simulink model "Vehicle10DOF"  (R2026b)
settings: Solver=ode45  StopTime=1
undefined symbols (not defined in the file): Tire, Vehicle, Vehicle7DOFInitialState
settings Model: DataDictionary=VehicleData.sldd  Creator=Xu Dingyi  LastModifiedBy=29358
settings ModelReferenceCC: ModelReferenceMinAlgLoopOccurrences=on

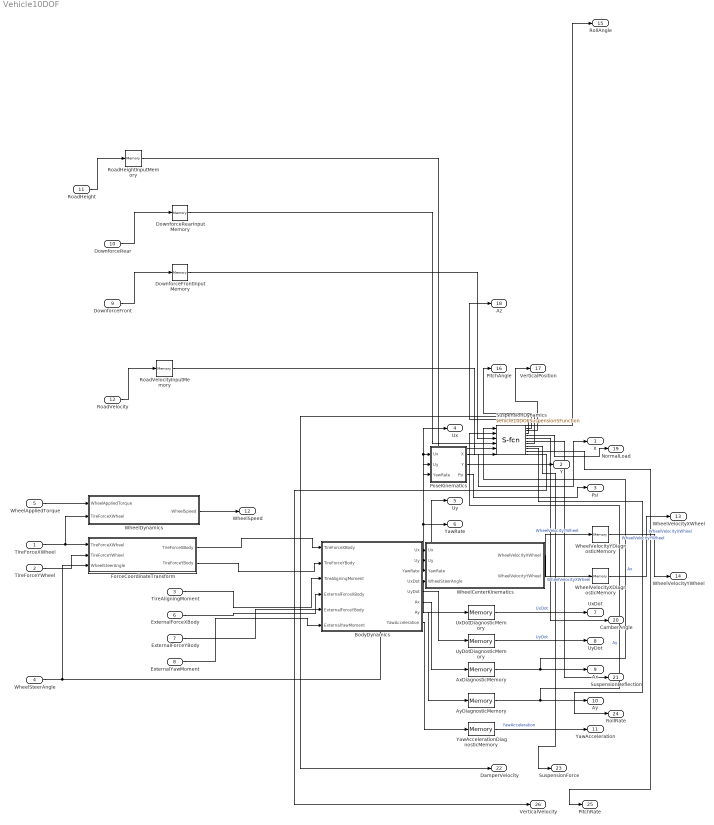
== system Vehicle10DOF ==
  TireForceXWheel : Inport  OutDataTypeStr=double  PortDimensions=[4 1]
  TireForceYWheel : Inport  Port=2  OutDataTypeStr=double  PortDimensions=[4 1]
  TireAligningMoment : Inport  Port=3  OutDataTypeStr=double  PortDimensions=[4 1]
  WheelSteerAngle : Inport  Port=4  OutDataTypeStr=double  PortDimensions=[4 1]
  WheelAppliedTorque : Inport  Port=5  OutDataTypeStr=double  PortDimensions=[4 1]
  ExternalForceXBody : Inport  Port=6  OutDataTypeStr=double  PortDimensions=1
  ExternalForceYBody : Inport  Port=7  OutDataTypeStr=double  PortDimensions=1
  ExternalYawMoment : Inport  Port=8  OutDataTypeStr=double  PortDimensions=1
  DownforceFront : Inport  Port=9
  DownforceRear : Inport  Port=10
  RoadHeight : Inport  Port=11  PortDimensions=4
  RoadVelocity : Inport  Port=12  PortDimensions=4
  AxDiagnosticMemory : Memory
  AyDiagnosticMemory : Memory
  BodyDynamics : Subsystem
  DownforceFrontInputMemory : Memory
  DownforceRearInputMemory : Memory
  ForceCoordinateTransform : Subsystem
  PoseKinematics : Subsystem
  RoadHeightInputMemory : Memory
  RoadVelocityInputMemory : Memory
  SuspensionDynamics : M-S-Function  FunctionName=vehicle10DOFSuspensionSFunction  Parameters=Vehicle10DOFSuspension
  UxDotDiagnosticMemory : Memory
  UyDotDiagnosticMemory : Memory
  WheelCenterKinematics : Subsystem
  WheelDynamics : Subsystem
  WheelVelocityXDiagnosticMemory : Memory
  WheelVelocityYDiagnosticMemory : Memory
  YawAccelerationDiagnosticMemory : Memory
  X : Outport
  Y : Outport  Port=2
  Psi : Outport  Port=3
  Ux : Outport  Port=4
  Uy : Outport  Port=5
  YawRate : Outport  Port=6
  UxDot : Outport  Port=7
  UyDot : Outport  Port=8
  Ax : Outport  Port=9
  Ay : Outport  Port=10
  YawAcceleration : Outport  Port=11
  WheelSpeed : Outport  Port=12
  WheelVelocityXWheel : Outport  Port=13
  WheelVelocityYWheel : Outport  Port=14
  RollAngle : Outport  Port=15
  PitchAngle : Outport  Port=16
  VerticalPosition : Outport  Port=17
  Az : Outport  Port=18
  NormalLoad : Outport  Port=19
  CamberAngle : Outport  Port=20
  SuspensionDeflection : Outport  Port=21
  DamperVelocity : Outport  Port=22
  SuspensionForce : Outport  Port=23
  RollRate : Outport  Port=24
  PitchRate : Outport  Port=25
  VerticalVelocity : Outport  Port=26
  wires:
  WheelSteerAngle/1 -> WheelCenterKinematics/4(WheelSteerAngle), ForceCoordinateTransform/3(WheelSteerAngle)
  TireForceYWheel/1 -> ForceCoordinateTransform/2(TireForceYWheel)
  TireForceXWheel/1 -> ForceCoordinateTransform/1(TireForceXWheel), WheelDynamics/2(TireForceXWheel)
  WheelAppliedTorque/1 -> WheelDynamics/1(WheelAppliedTorque)
  YawAccelerationDiagnosticMemory/1 -> YawAcceleration/1  "YawAcceleration"
  WheelDynamics/1(WheelSpeed) -> WheelSpeed/1
  UxDotDiagnosticMemory/1 -> UxDot/1  "UxDot"
  UyDotDiagnosticMemory/1 -> UyDot/1  "UyDot"
  AyDiagnosticMemory/1 -> SuspensionDynamics/2, Ay/1  "Ay"
  ForceCoordinateTransform/1(TireForceXBody) -> BodyDynamics/1(TireForceXBody)
  ForceCoordinateTransform/2(TireForceYBody) -> BodyDynamics/2(TireForceYBody)
  TireAligningMoment/1 -> BodyDynamics/3(TireAligningMoment)
  ExternalForceXBody/1 -> BodyDynamics/4(ExternalForceXBody)
  ExternalForceYBody/1 -> BodyDynamics/5(ExternalForceYBody)
  ExternalYawMoment/1 -> BodyDynamics/6(ExternalYawMoment)
  BodyDynamics/4(UxDot) -> UxDotDiagnosticMemory/1
  BodyDynamics/5(UyDot) -> UyDotDiagnosticMemory/1
  BodyDynamics/6(Ax) -> AxDiagnosticMemory/1
  BodyDynamics/7(Ay) -> AyDiagnosticMemory/1
  BodyDynamics/8(YawAcceleration) -> YawAccelerationDiagnosticMemory/1
  AxDiagnosticMemory/1 -> SuspensionDynamics/1, Ax/1  "Ax"
  BodyDynamics/1(Ux) -> Ux/1, PoseKinematics/1(Ux), WheelCenterKinematics/1(Ux)
  BodyDynamics/2(Uy) -> PoseKinematics/2(Uy), Uy/1, WheelCenterKinematics/2(Uy)
  BodyDynamics/3(YawRate) -> PoseKinematics/3(YawRate), YawRate/1, WheelCenterKinematics/3(YawRate)
  PoseKinematics/1(X) -> X/1
  PoseKinematics/2(Y) -> Y/1
  PoseKinematics/3(Psi) -> Psi/1
  WheelCenterKinematics/1(WheelVelocityXWheel) -> WheelVelocityXDiagnosticMemory/1  "WheelVelocityXWheel"
  WheelVelocityXDiagnosticMemory/1 -> WheelVelocityXWheel/1  "WheelVelocityXWheel"
  WheelCenterKinematics/2(WheelVelocityYWheel) -> WheelVelocityYDiagnosticMemory/1  "WheelVelocityYWheel"
  WheelVelocityYDiagnosticMemory/1 -> WheelVelocityYWheel/1  "WheelVelocityYWheel"
  DownforceFront/1 -> DownforceFrontInputMemory/1
  DownforceRear/1 -> DownforceRearInputMemory/1
  RoadHeight/1 -> RoadHeightInputMemory/1
  RoadVelocity/1 -> RoadVelocityInputMemory/1
  SuspensionDynamics/1 -> RollAngle/1
  SuspensionDynamics/2 -> PitchAngle/1
  SuspensionDynamics/3 -> VerticalPosition/1
  SuspensionDynamics/4 -> Az/1
  SuspensionDynamics/5 -> NormalLoad/1
  SuspensionDynamics/6 -> CamberAngle/1
  SuspensionDynamics/7 -> SuspensionDeflection/1
  SuspensionDynamics/8 -> DamperVelocity/1
  SuspensionDynamics/9 -> SuspensionForce/1
  SuspensionDynamics/10 -> RollRate/1
  SuspensionDynamics/11 -> PitchRate/1
  SuspensionDynamics/12 -> VerticalVelocity/1
  DownforceFrontInputMemory/1 -> SuspensionDynamics/3
  DownforceRearInputMemory/1 -> SuspensionDynamics/4
  RoadHeightInputMemory/1 -> SuspensionDynamics/5
  RoadVelocityInputMemory/1 -> SuspensionDynamics/6

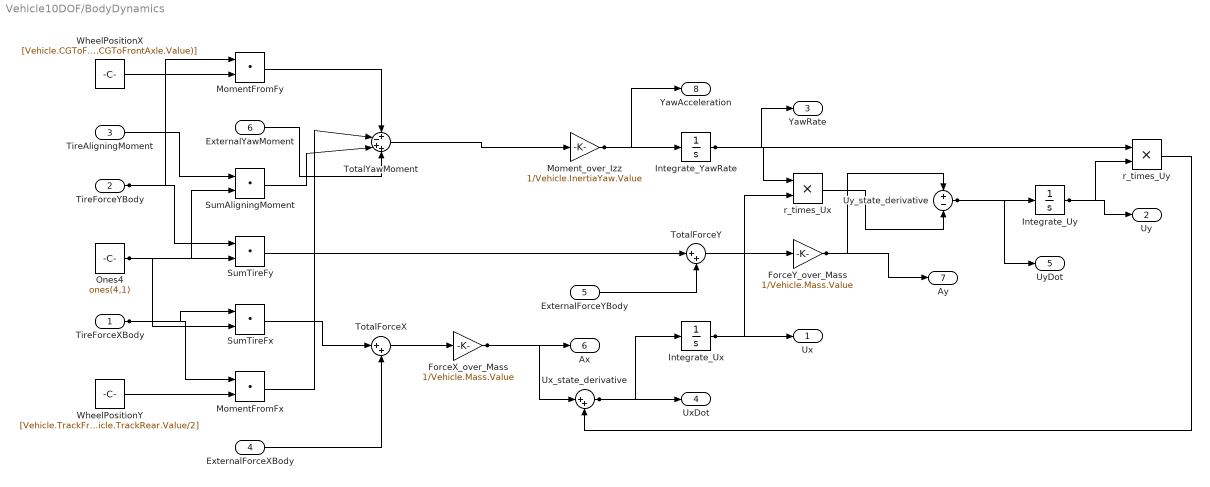
== system Vehicle10DOF/BodyDynamics ==
  TireForceXBody : Inport
  TireForceYBody : Inport  Port=2
  TireAligningMoment : Inport  Port=3
  ExternalForceXBody : Inport  Port=4
  ExternalForceYBody : Inport  Port=5
  ExternalYawMoment : Inport  Port=6
  ForceX_over_Mass : Gain  Gain=1/Vehicle.Mass.Value
  ForceY_over_Mass : Gain  Gain=1/Vehicle.Mass.Value
  Integrate_Ux : Integrator  InitialCondition=Vehicle7DOFInitialState.Ux
  Integrate_Uy : Integrator  InitialCondition=Vehicle7DOFInitialState.Uy
  Integrate_YawRate : Integrator  InitialCondition=Vehicle7DOFInitialState.YawRate
  MomentFromFx : DotProduct
  MomentFromFy : DotProduct
  Moment_over_Izz : Gain  Gain=1/Vehicle.InertiaYaw.Value
  Ones4 : Constant  Value=ones(4,1)  OutDataTypeStr=double
  SumAligningMoment : DotProduct
  SumTireFx : DotProduct
  SumTireFy : DotProduct
  TotalForceX : Sum  Inputs=|++
  TotalForceY : Sum  Inputs=|++
  TotalYawMoment : Sum  Inputs=+-++
  Ux_state_derivative : Sum  Inputs=|++
  Uy_state_derivative : Sum  Inputs=+-
  WheelPositionX : Constant  Value=[Vehicle.CGToFrontAxle.Value; Vehicle.CGToFrontAxle.Value; -(Vehicle.Wheelbase.Value-Vehicle.CGToFrontAxle.Value); -(Vehicle.Wheelbase.Value-Vehicle.CGToFrontAxle.Value)]  OutDataTypeStr=double
  WheelPositionY : Constant  Value=[Vehicle.TrackFront.Value/2; -Vehicle.TrackFront.Value/2; Vehicle.TrackRear.Value/2; -Vehicle.TrackRear.Value/2]  OutDataTypeStr=double
  r_times_Ux : Product  Inputs=**
  r_times_Uy : Product  Inputs=**
  Ux : Outport
  Uy : Outport  Port=2
  YawRate : Outport  Port=3
  UxDot : Outport  Port=4
  UyDot : Outport  Port=5
  Ax : Outport  Port=6
  Ay : Outport  Port=7
  YawAcceleration : Outport  Port=8
  wires:
  Moment_over_Izz/1 -> Integrate_YawRate/1, YawAcceleration/1
  Uy_state_derivative/1 -> Integrate_Uy/1, UyDot/1
  Ux_state_derivative/1 -> Integrate_Ux/1, UxDot/1
  r_times_Ux/1 -> Uy_state_derivative/2
  ForceY_over_Mass/1 -> Uy_state_derivative/1, Ay/1
  r_times_Uy/1 -> Ux_state_derivative/2
  ForceX_over_Mass/1 -> Ux_state_derivative/1, Ax/1
  Integrate_Ux/1 -> r_times_Ux/2, Ux/1
  Integrate_Uy/1 -> r_times_Uy/2, Uy/1
  Integrate_YawRate/1 -> r_times_Uy/1, r_times_Ux/1, YawRate/1
  TotalYawMoment/1 -> Moment_over_Izz/1
  TotalForceY/1 -> ForceY_over_Mass/1
  TotalForceX/1 -> ForceX_over_Mass/1
  ExternalYawMoment/1 -> TotalYawMoment/4
  SumAligningMoment/1 -> TotalYawMoment/3
  MomentFromFx/1 -> TotalYawMoment/2
  MomentFromFy/1 -> TotalYawMoment/1
  ExternalForceYBody/1 -> TotalForceY/2
  SumTireFy/1 -> TotalForceY/1
  ExternalForceXBody/1 -> TotalForceX/2
  SumTireFx/1 -> TotalForceX/1
  TireAligningMoment/1 -> SumAligningMoment/1
  WheelPositionY/1 -> MomentFromFx/2
  WheelPositionX/1 -> MomentFromFy/2
  TireForceYBody/1 -> SumTireFy/1, MomentFromFy/1
  Ones4/1 -> SumTireFx/2, SumTireFy/2, SumAligningMoment/2
  TireForceXBody/1 -> SumTireFx/1, MomentFromFx/1

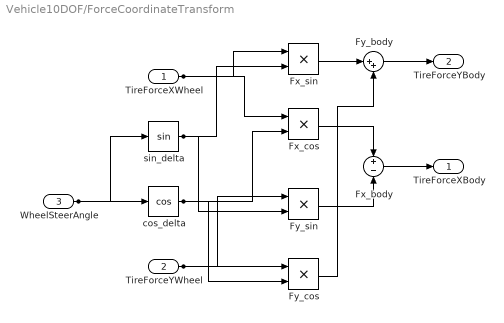
== system Vehicle10DOF/ForceCoordinateTransform ==
  TireForceXWheel : Inport
  TireForceYWheel : Inport  Port=2
  WheelSteerAngle : Inport  Port=3
  Fx_body : Sum  Inputs=+-
  Fx_cos : Product  Inputs=**
  Fx_sin : Product  Inputs=**
  Fy_body : Sum  Inputs=|++
  Fy_cos : Product  Inputs=**
  Fy_sin : Product  Inputs=**
  cos_delta : Trigonometry  Operator=cos
  sin_delta : Trigonometry
  TireForceXBody : Outport
  TireForceYBody : Outport  Port=2
  wires:
  Fy_body/1 -> TireForceYBody/1
  Fx_body/1 -> TireForceXBody/1
  Fy_cos/1 -> Fy_body/2
  Fx_sin/1 -> Fy_body/1
  Fy_sin/1 -> Fx_body/2
  Fx_cos/1 -> Fx_body/1
  sin_delta/1 -> Fy_sin/2, Fx_sin/2
  TireForceYWheel/1 -> Fy_sin/1, Fy_cos/1
  cos_delta/1 -> Fx_cos/2, Fy_cos/2
  TireForceXWheel/1 -> Fx_cos/1, Fx_sin/1
  WheelSteerAngle/1 -> cos_delta/1, sin_delta/1

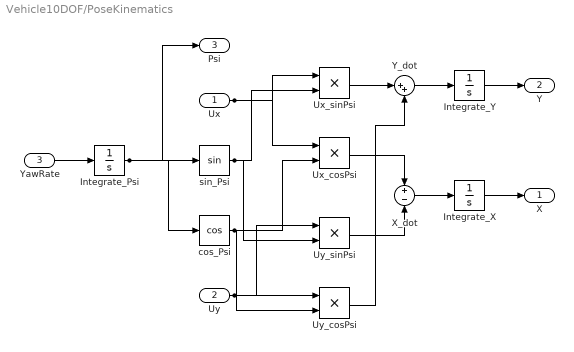
== system Vehicle10DOF/PoseKinematics ==
  Ux : Inport
  Uy : Inport  Port=2
  YawRate : Inport  Port=3
  Integrate_Psi : Integrator  InitialCondition=Vehicle7DOFInitialState.Psi
  Integrate_X : Integrator  InitialCondition=Vehicle7DOFInitialState.X
  Integrate_Y : Integrator  InitialCondition=Vehicle7DOFInitialState.Y
  Ux_cosPsi : Product  Inputs=**
  Ux_sinPsi : Product  Inputs=**
  Uy_cosPsi : Product  Inputs=**
  Uy_sinPsi : Product  Inputs=**
  X_dot : Sum  Inputs=+-
  Y_dot : Sum  Inputs=|++
  cos_Psi : Trigonometry  Operator=cos
  sin_Psi : Trigonometry
  X : Outport
  Y : Outport  Port=2
  Psi : Outport  Port=3
  wires:
  Integrate_Y/1 -> Y/1
  Integrate_X/1 -> X/1
  YawRate/1 -> Integrate_Psi/1
  Y_dot/1 -> Integrate_Y/1
  X_dot/1 -> Integrate_X/1
  Uy_cosPsi/1 -> Y_dot/2
  Ux_sinPsi/1 -> Y_dot/1
  Uy_sinPsi/1 -> X_dot/2
  Ux_cosPsi/1 -> X_dot/1
  sin_Psi/1 -> Uy_sinPsi/2, Ux_sinPsi/2
  Uy/1 -> Uy_sinPsi/1, Uy_cosPsi/1
  cos_Psi/1 -> Ux_cosPsi/2, Uy_cosPsi/2
  Ux/1 -> Ux_cosPsi/1, Ux_sinPsi/1
  Integrate_Psi/1 -> cos_Psi/1, sin_Psi/1, Psi/1

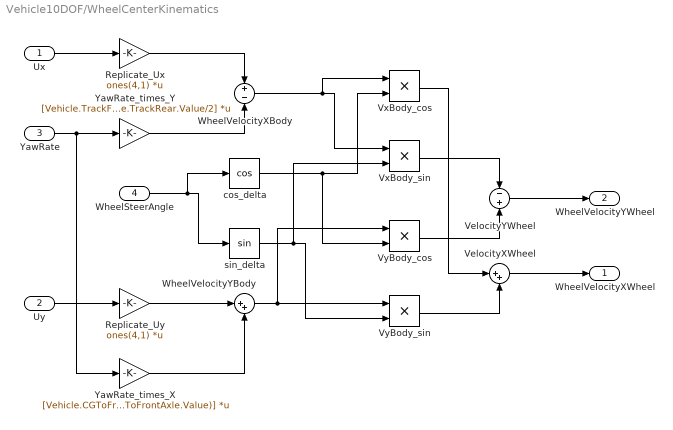
== system Vehicle10DOF/WheelCenterKinematics ==
  Ux : Inport
  Uy : Inport  Port=2
  YawRate : Inport  Port=3
  WheelSteerAngle : Inport  Port=4
  Replicate_Ux : Gain  Gain=ones(4,1)  Multiplication=Matrix(K*u)
  Replicate_Uy : Gain  Gain=ones(4,1)  Multiplication=Matrix(K*u)
  VelocityXWheel : Sum  Inputs=|++
  VelocityYWheel : Sum  Inputs=-+
  VxBody_cos : Product  Inputs=**
  VxBody_sin : Product  Inputs=**
  VyBody_cos : Product  Inputs=**
  VyBody_sin : Product  Inputs=**
  WheelVelocityXBody : Sum  Inputs=+-
  WheelVelocityYBody : Sum  Inputs=|++
  YawRate_times_X : Gain  Gain=[Vehicle.CGToFrontAxle.Value; Vehicle.CGToFrontAxle.Value; -(Vehicle.Wheelbase.Value-Vehicle.CGToFrontAxle.Value); -(Vehicle.Wheelbase.Value-Vehicle.CGToFrontAxle.Value)]  Multiplication=Matrix(K*u)
  YawRate_times_Y : Gain  Gain=[Vehicle.TrackFront.Value/2; -Vehicle.TrackFront.Value/2; Vehicle.TrackRear.Value/2; -Vehicle.TrackRear.Value/2]  Multiplication=Matrix(K*u)
  cos_delta : Trigonometry  Operator=cos
  sin_delta : Trigonometry
  WheelVelocityXWheel : Outport
  WheelVelocityYWheel : Outport  Port=2
  wires:
  VelocityYWheel/1 -> WheelVelocityYWheel/1
  VelocityXWheel/1 -> WheelVelocityXWheel/1
  VyBody_cos/1 -> VelocityYWheel/2
  VxBody_sin/1 -> VelocityYWheel/1
  VyBody_sin/1 -> VelocityXWheel/2
  VxBody_cos/1 -> VelocityXWheel/1
  sin_delta/1 -> VyBody_sin/2, VxBody_sin/2
  WheelVelocityYBody/1 -> VyBody_sin/1, VyBody_cos/1
  cos_delta/1 -> VxBody_cos/2, VyBody_cos/2
  WheelVelocityXBody/1 -> VxBody_cos/1, VxBody_sin/1
  WheelSteerAngle/1 -> cos_delta/1, sin_delta/1
  YawRate_times_X/1 -> WheelVelocityYBody/2
  Replicate_Uy/1 -> WheelVelocityYBody/1
  YawRate_times_Y/1 -> WheelVelocityXBody/2
  Replicate_Ux/1 -> WheelVelocityXBody/1
  YawRate/1 -> YawRate_times_Y/1, YawRate_times_X/1
  Uy/1 -> Replicate_Uy/1
  Ux/1 -> Replicate_Ux/1

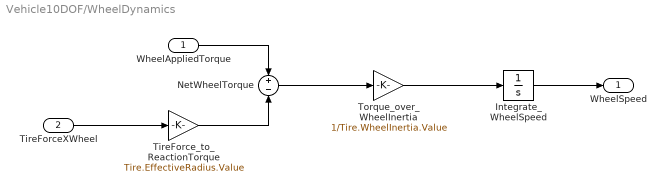
== system Vehicle10DOF/WheelDynamics ==
  WheelAppliedTorque : Inport
  TireForceXWheel : Inport  Port=2
  Integrate_WheelSpeed : Integrator  InitialCondition=Vehicle7DOFInitialState.WheelSpeed
  NetWheelTorque : Sum  Inputs=+-
  TireForce_to_ReactionTorque : Gain  Gain=Tire.EffectiveRadius.Value
  Torque_over_WheelInertia : Gain  Gain=1/Tire.WheelInertia.Value
  WheelSpeed : Outport
  wires:
  Integrate_WheelSpeed/1 -> WheelSpeed/1
  Torque_over_WheelInertia/1 -> Integrate_WheelSpeed/1
  NetWheelTorque/1 -> Torque_over_WheelInertia/1
  TireForce_to_ReactionTorque/1 -> NetWheelTorque/2
  WheelAppliedTorque/1 -> NetWheelTorque/1
  TireForceXWheel/1 -> TireForce_to_ReactionTorque/1
